simulink model "CANTxRxManager"  (R2024a)
settings: Solver=VariableStepAuto  StartTime=0.0  StopTime=10.0  RelTol=1e-3
undefined symbols (not defined in the file): maxCurrent_A, maxVoltage_V, powerRequest_kW, VCU_Request_IF
settings Model: DataDictionary=BMS_System_Arch_dict.sldd  Creator=ghourabi  LastModifiedBy=ghourabi

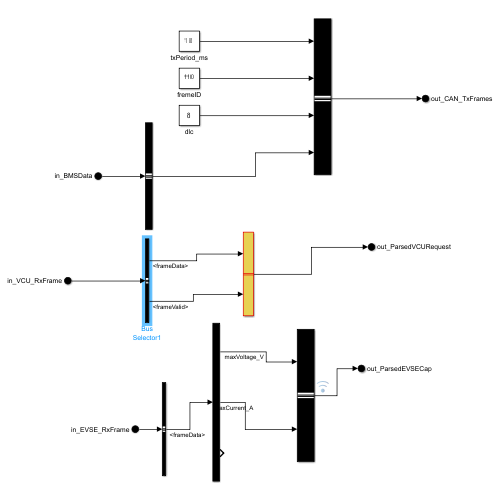
[thumbnail: Simulink's stored preview of the top-level diagram]
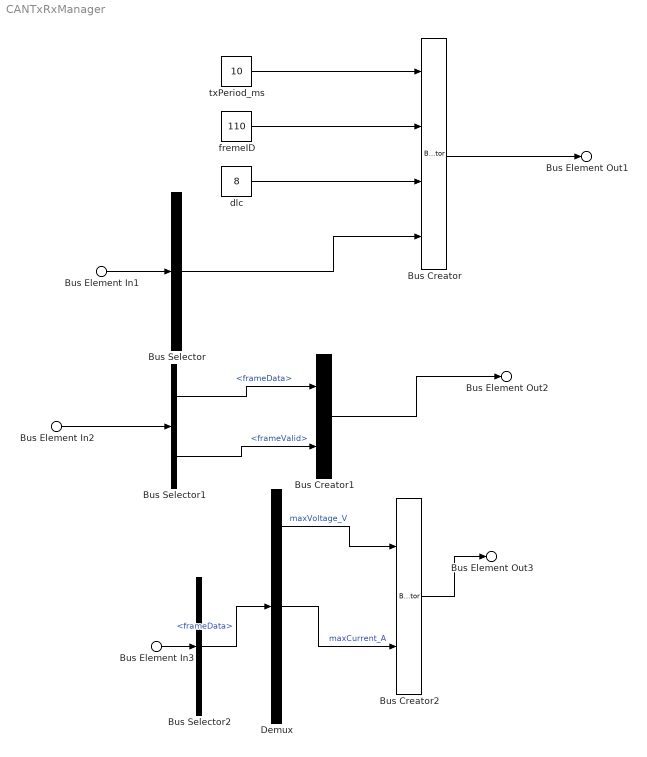
== system CANTxRxManager ==
  Bus Element In1 : Inport  PortName=in_BMSData
  Bus Element In2 : Inport  Port=2  PortName=in_VCU_RxFrame
  Bus Element In3 : Inport  Port=3  PortName=in_EVSE_RxFrame
  Bus Creator : BusCreator  Inputs=4
  Bus Creator1 : BusCreator  Inputs=VCU_Request_IF,powerRequest_kW  OutDataTypeStr=Bus: VCU_Request_IF
  Bus Creator2 : BusCreator  Inputs=maxVoltage_V,maxCurrent_A  OutDataTypeStr=Bus: EVSE_Cap_IF
  Bus Selector : BusSelector  OutputSignals=packVoltage,sopDischarge,sopCharge,tempMin,tempMax,packCurrent,soc  OutputAsBus=on
  Bus Selector1 : BusSelector  OutputSignals=frameData,frameValid
  Bus Selector2 : BusSelector  OutputSignals=frameData
  Demux : Demux  Outputs=3
  dlc : Constant  Value=8
  fremeID : Constant  Value=110
  txPeriod_ms : Constant  Value=10
  Bus Element Out1 : Outport  PortName=out_CAN_TxFrames
  Bus Element Out2 : Outport  Port=2  PortName=out_ParsedVCURequest
  Bus Element Out3 : Outport  Port=3  PortName=out_ParsedEVSECap
  wires:
  Bus Element In1/1 -> Bus Selector/1
  Bus Selector/1 -> Bus Creator/4
  txPeriod_ms/1 -> Bus Creator/1
  fremeID/1 -> Bus Creator/2
  dlc/1 -> Bus Creator/3
  Bus Creator/1 -> Bus Element Out1/1
  Bus Element In2/1 -> Bus Selector1/1
  Bus Selector1/1 -> Bus Creator1/1  "<frameData>"
  Bus Selector1/2 -> Bus Creator1/2  "<frameValid>"
  Bus Creator1/1 -> Bus Element Out2/1
  Bus Creator2/1 -> Bus Element Out3/1
  Bus Element In3/1 -> Bus Selector2/1
  Bus Selector2/1 -> Demux/1  "<frameData>"
  Demux/1 -> Bus Creator2/1  "maxVoltage_V"
  Demux/2 -> Bus Creator2/2  "maxCurrent_A"
